simulink model "q8b"  (R2014a)
settings: Solver=ode45  StartTime=0.0  StopTime=10  RelTol=1e-3
settings Model: Creator=Primarch-IV  LastModifiedBy=Primarch-IV

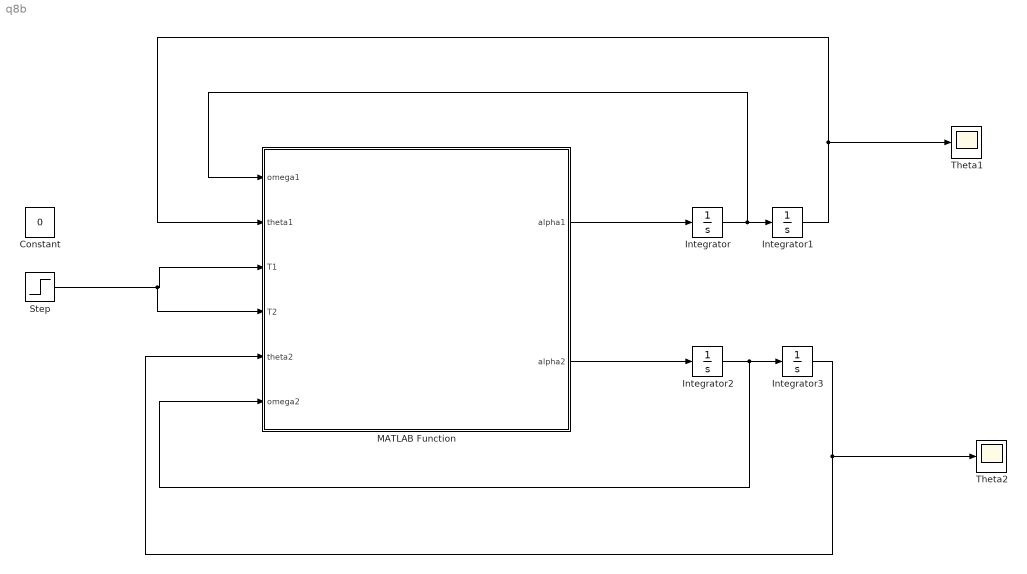
== system q8b ==
  Constant : Constant  Value=0
  Integrator{,1..3} (4 alike) : Integrator
  MATLAB Function : MATLAB Function  TreatAsAtomicUnit=on
  Step : Step  SampleTime=0
  Theta1 : Scope
      settings: YMin=-100  YMax=0
  Theta2 : Scope
  wires:
  MATLAB Function/2(alpha2) -> Integrator2/1
  Integrator2/1 -> Integrator3/1, MATLAB Function/6(omega2)
  Integrator3/1 -> MATLAB Function/5(theta2), Theta2/1
  MATLAB Function/1(alpha1) -> Integrator/1
  Integrator/1 -> Integrator1/1, MATLAB Function/1(omega1)
  Integrator1/1 -> Theta1/1, MATLAB Function/2(theta1)
  Step/1 -> MATLAB Function/4(T2), MATLAB Function/3(T1)

== matlab function q8b/MATLAB Function ==
  data: omega1 input; alpha1 output; theta1 input; T1 input; T2 input; theta2 input; omega2 input; alpha2 output
function [alpha1,alpha2] = fcn(omega1,theta1,T1,T2,theta2,omega2)
%#codegen

% Torque 1&2
% syms T1
% syms T2
% Angles 1&2
% syms theta1
% syms theta2
% Angular Velocity 1&2
% syms omega1
% syms omega2
% Angular Acceleration 1&2
% syms alpha1
% syms alpha2
% 
% Acceleration due to Gravity
% g = 9.8;

%alpha1 = (T1 - alpha2*(0.7625 + 1.5*cos(theta2)) + omega1*omega2*(3*sin(theta2)) + omega2*3*sin(theta2) - 6.5*g*cos(theta1) + 1.5*g*cos(theta1 + theta2))/(5.1625 + 3*cos(theta2));
%alpha2 = (T2 - alpha1*(0.7625 + 1.5*cos(theta2) - omega1^2*(1.5*sin(theta2))) - 1.5*g*cos(theta1 + theta2))/0.2;
% s = solve(alpha1 == (T1 - alpha2*(0.7625 + 1.5*cos(theta2)) + omega1*omega2*(3*sin(theta2)) + omega2*3*sin(theta2) - 6.5*g*cos(theta1) + 1.5*g*cos(theta1 + theta2))/(5.1625 + 3*cos(theta2)),alpha2 == (T2 - alpha1*(0.7625 + 1.5*cos(theta2) - omega1^2*(1.5*sin(theta2))) - 1.5*g*cos(theta1 + theta2))/0.2 ,alpha1,alpha2);

% alpha1 = s.alpha1;
% alpha2 = s.alpha2;

% alpha1 = (2*(3200*T1 - 12200*T2 + 226611*cos(theta1 + theta2) - 204048*cos(theta1) - 24000*T2*cos(theta2) + 9600*omega2*sin(theta2) + 353160*cos(theta1 + theta2)*cos(theta2) + 9600*omega1*omega2*sin(theta2)))/(5*(7320*omega1^2*sin(theta2) - 10800*cos(theta2) - 14400*cos(theta2)^2 + 14400*omega1^2*cos(theta2)*sin(theta2) + 2887));
% alpha2 = -(2*(12200*T1 - 82600*T2 + 1394982*cos(theta1 + theta2) - 777933*cos(theta1) - 1530360*cos(theta1)*cos(theta2) + 24000*T1*cos(theta2) - 48000*T2*cos(theta2) + 36600*omega2*sin(theta2) + 1059480*cos(theta1 + theta2)*cos(theta2) + 36600*omega1*omega2*sin(theta2) - 24000*T1*omega1^2*sin(theta2) + 72000*omega2*cos(theta2)*sin(theta2) - 353160*omega1^2*cos(theta1 + theta2)*sin(theta2) - 72000*omega1^2*omega2*sin(theta2)^2 - 72000*omega1^3*omega2*sin(theta2)^2 + 1530360*omega1^2*cos(theta1)*sin(theta2) + 72000*omega1*omega2*cos(theta2)*sin(theta2)))/(5*(7320*omega1^2*sin(theta2) - 10800*cos(theta2) - 14400*cos(theta2)^2 + 14400*omega1^2*cos(theta2)*sin(theta2) + 2887));

 
alpha1 = (8*(160*T1 - 610*T2 + 11319*cos(theta1 + theta2) - 10192*cos(theta1) - 1200*T2*cos(theta2) + 480*omega2*sin(theta2) + 17640*cos(theta1 + theta2)*cos(theta2) + 480*omega1*omega2*sin(theta2)))/(7320*omega1^2*sin(theta2) - 10800*cos(theta2) - 14400*cos(theta2)^2 + 14400*omega1^2*cos(theta2)*sin(theta2) + 2887);
alpha2 = -(8*(610*T1 - 4130*T2 + 69678*cos(theta1 + theta2) - 38857*cos(theta1) - 76440*cos(theta1)*cos(theta2) + 1200*T1*cos(theta2) - 2400*T2*cos(theta2) + 1830*omega2*sin(theta2) + 52920*cos(theta1 + theta2)*cos(theta2) + 1830*omega1*omega2*sin(theta2) - 1200*T1*omega1^2*sin(theta2) + 3600*omega2*cos(theta2)*sin(theta2) - 17640*omega1^2*cos(theta1 + theta2)*sin(theta2) - 3600*omega1^2*omega2*sin(theta2)^2 - 3600*omega1^3*omega2*sin(theta2)^2 + 76440*omega1^2*cos(theta1)*sin(theta2) + 3600*omega1*omega2*cos(theta2)*sin(theta2)))/(7320*omega1^2*sin(theta2) - 10800*cos(theta2) - 14400*cos(theta2)^2 + 14400*omega1^2*cos(theta2)*sin(theta2) + 2887);
